simulink model "non_linear_v2"  (R2019a)
settings: Solver=VariableStepAuto  StartTime=0.0  StopTime=10  RelTol=1e-3
values from neighbouring files (symbols this model uses):
  K = lqr(linA,linB,Q,R)    [controller.m]
settings Model: Creator=iyengar  LastModifiedBy=iyengar

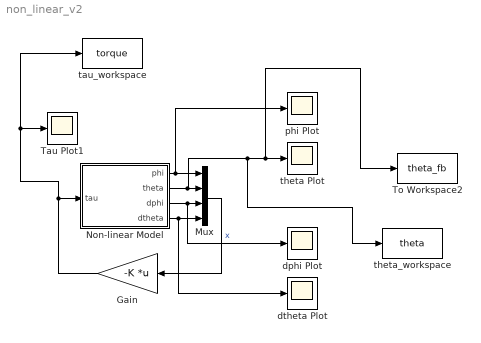
== system non_linear_v2 ==
  Gain : Gain  Gain=-K  Multiplication=Matrix(K*u)
  Mux : Mux
  Non-linear Model : Subsystem
  Tau Plot1 : Scope
  To Workspace2 : ToWorkspace  VariableName=theta_fb  SaveFormat=Timeseries  SampleTime=-1
  dphi Plot : Scope
  dtheta Plot : Scope
  phi Plot : Scope
  "tau_workspace " : ToWorkspace  VariableName=torque  SaveFormat=Timeseries  SampleTime=-1
  theta Plot : Scope
  "theta_workspace " : ToWorkspace  VariableName=theta  SaveFormat=Timeseries  SampleTime=-1
  wires:
  Gain/1 -> "tau_workspace "/1, Tau Plot1/1, Non-linear Model/1(tau)
  Non-linear Model/1(phi) -> phi Plot/1, Mux/1
  Non-linear Model/2(theta) -> "theta_workspace "/1, To Workspace2/1, theta Plot/1, Mux/2
  Non-linear Model/3(dphi) -> dphi Plot/1, Mux/3
  Non-linear Model/4(dtheta) -> dtheta Plot/1, Mux/4
  Mux/1 -> Gain/1  "x"

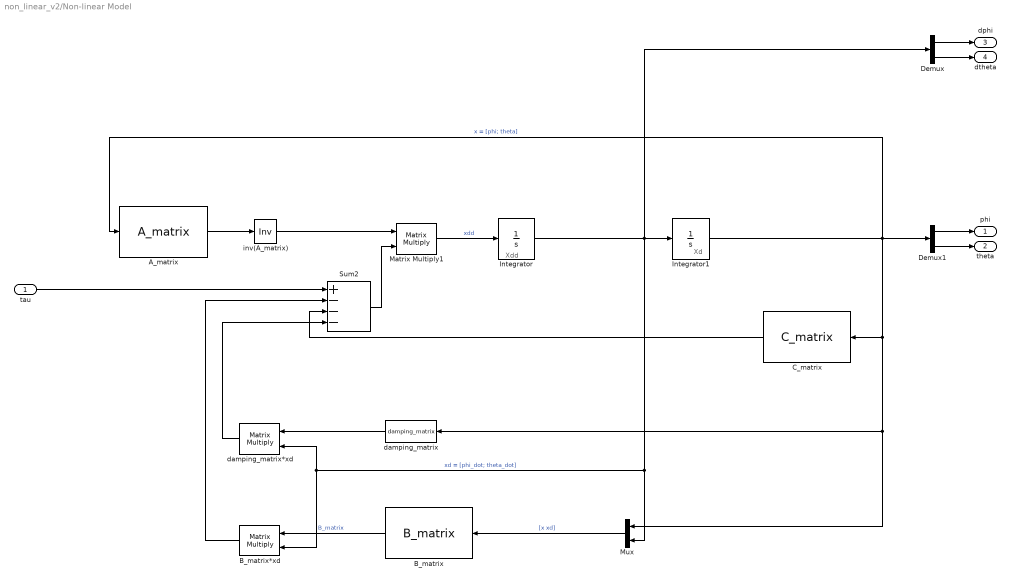
== system non_linear_v2/Non-linear Model ==
  note: Xdd
  note: Xd
  tau : Inport
  "A_matrix " : MATLABFcn  Description=matrix A. 2x2  MATLABFcn=A_matrix  Output1D=off
  B_matrix : MATLABFcn  MATLABFcn=B_matrix  Output1D=off
  B_matrix*xd : Product  Multiplication=Matrix(*)
  C_matrix : MATLABFcn  MATLABFcn=C_matrix  OutputDimensions=2  Output1D=off
  Demux : Demux  Outputs=2
  Demux1 : Demux  Outputs=2
  Integrator : Integrator  InitialCondition=[0; 0.5]
  Integrator1 : Integrator  InitialCondition=[0; 0.05]
  Matrix Multiply1 : Product  Multiplication=Matrix(*)
  Mux : Mux  Inputs=2
  Sum2 : Sum  Inputs=+---
  damping_matrix : MATLABFcn  MATLABFcn=damping_matrix  Output1D=off
  "damping_matrix*xd " : Product  Multiplication=Matrix(*)
  inv(A_matrix) : Product  Inputs=/  Multiplication=Matrix(*)
  phi : Outport
  theta : Outport  Port=2
  dphi : Outport  Port=3
  dtheta : Outport  Port=4
  wires:
  Mux/1 -> B_matrix/1  "[x xd]"
  Demux/2 -> dtheta/1
  Integrator/1 -> Demux/1, Integrator1/1, Mux/2, "damping_matrix*xd "/2, B_matrix*xd/2  "xd = [phi_dot; theta_dot]"
  Sum2/1 -> Matrix Multiply1/2
  C_matrix/1 -> Sum2/3
  Demux1/2 -> theta/1
  Integrator1/1 -> Demux1/1, "A_matrix "/1, damping_matrix/1, Mux/1, C_matrix/1  "x = [phi; theta]"
  Matrix Multiply1/1 -> Integrator/1  "xdd"
  "damping_matrix*xd "/1 -> Sum2/4
  B_matrix*xd/1 -> Sum2/2
  B_matrix/1 -> B_matrix*xd/1  "B_matrix"
  inv(A_matrix)/1 -> Matrix Multiply1/1
  "A_matrix "/1 -> inv(A_matrix)/1
  damping_matrix/1 -> "damping_matrix*xd "/1
  tau/1 -> Sum2/1
  Demux/1 -> dphi/1
  Demux1/1 -> phi/1
